simulink model "RealSimTemplate"  (R2019b)
settings: Solver=FixedStepAuto  StartTime=0.0  StopTime=200  FixedStep=0.001  RelTol=1e-3
settings Model: Creator=y0n  LastModifiedBy=y0n
settings DataIOCC: SaveOutput=off  SignalLogging=off  DSMLogging=off  SaveTime=off  ReturnWorkspaceOutputsName=VehicleOut
settings DebuggingCC: AlgebraicLoopMsg=none  UnderSpecifiedDimensionMsg=error
settings SFSimCC: CustomCodeUndefinedFunction=UseInterfaceOnly

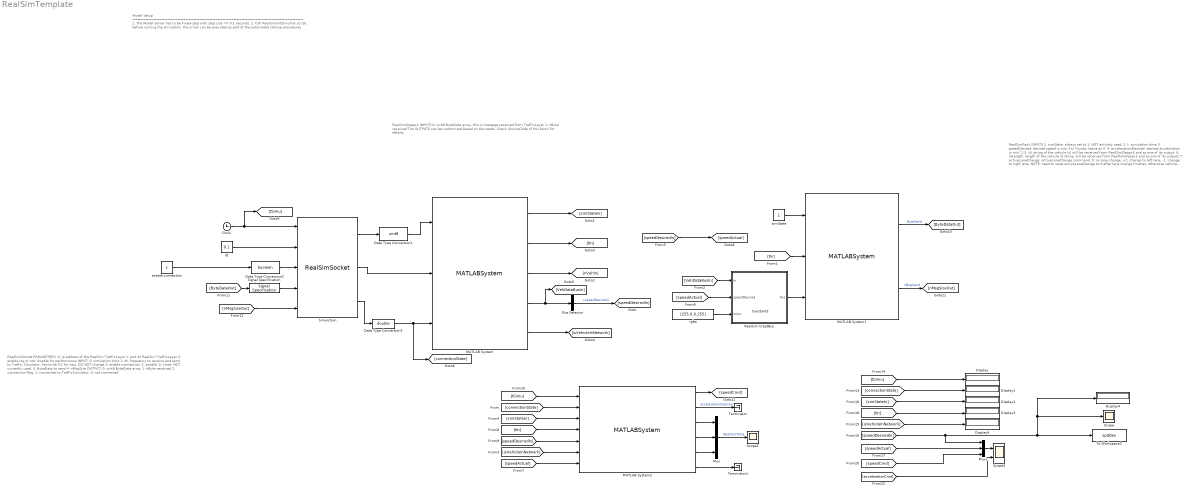
== system RealSimTemplate ==
  note: Model Setup
      | ================================================================
      | 1. The Model Solver has to be Fixed-step with step size <= 0.1 seconds.
      | 2. Call RealSimInitSimulink script before running the simulation. the script can be executed as part of the automated startup procedures.
  note: RealSimSocket
      | PARAMETERS:
      | 0: ip address of the RealSim TrafficLayer
      | 1: port to RealSim TrafficLayer
      | 2: enable log or not, disable for performance
      | INPUT:
      | 0: simulation time
      | 1: dt, frequency to receive and send to Traffic Simulator, has to be 0.1 for now, DO NOT change
      | 2: enable connection, 1: enable, 0: close. NOT currently used.
      | 3: ByteData to send
      | 4: nMsgSize
      |
      | OUTPUT:
      | 0: uint8 ByteData array
      | 1: nByte received
      | 2: connection flag, 1: connected to TrafficSimulator, 0: not connected
  note: RealSimPack
      | INPUTS
      | 1. simState: always set to 1. NOT actively used.
      | 2. t: simulation time
      | 3. speedDesired: desired speed in m/s, For Toyota, leave as 0.
      | 4. accelerationDesired: desired acceleration in m/s^2
      | 5. id: string of the vehicle id, will be received from RealSimDepack and as one of its output.
      | 6. idLength: length of the vehicle id string, will be received from RealSimDepack and as one of its outputs
      | 7: activeLaneChange: activeLaneChange command, 0: no lane change, +1: change to left lane, -1: change to right lane. NOTE: need to reset activeLaneChange to 0 after lane change finishes, otherwise vehicle will keep making lane change. Will receive 0 activeLaneChangeFdbk from RealSimDepack when lane change finishes.
      |
      | NOTE 1: Currently, only speedDesired and/or accelerationDesired can be sent to VISSIM/SUMO. The data format receive and send are the same so other mesage fields of the send data are irrelevant and can be set to empty or zero.
      |
      | NOTE 2: if select both speedDesired and accelerationDesired
      | in config.yaml, then only accelerationDesired will be used
      | to control vehicles in TrafficSimulator. if only one of
      | speedDesired and accelerationDesired selected in
      | config.yaml, then the one selected will be used for
      | control, the other input can be leave as 0.
      |
      | NOTE 3: for VISSIM, speedDesired or accelerationDesired will be the control command 0.2 seconds in the future.
      |
      | OUTPUTS
      | 1.ByteData: bytes vector that will be sent to TrafficSimualtor
      | 2.nMsgSize: size of bytes to be sent
  note: RealSimDepack
      | INPUTS
      | 0: uint8 ByteData array, this is message received from TrafficLayer
      | 1: nByte received
      |
      | The OUTPUTS can be customized based on the needs. Check SourceCode of this block for details.
  Bus Selector : BusSelector  OutputSignals=speedDesired
  Clock : Clock
  Constant3 : Constant  Value=0
  Data Type Conversion1 : DataTypeConversion  OutDataTypeStr=uint8
  Data Type Conversion2 : DataTypeConversion  OutDataTypeStr=boolean
  Data Type Conversion3 : DataTypeConversion  OutDataTypeStr=double
  Display{,1..4,6} (6 alike) : Display
  MATLAB System : MATLABSystem  System=RealSimDepack  OutputBusName=VehDataBus  VehicleMessageFieldDefInputVec=VehicleMessageFieldDefInputVec  SimulateUsing=Code generation
      mask Type: RealSimDepack
      mask Display:
      | disp('RealSimDepack');
      | port_label('input',1,'ByteData');
      | port_label('input',2,'nByte');
      | port_label('input',3,'connectionState');
      | port_label('output',1,'simState');
      | port_label('output',2,'t');
      | port_label('output',3,'nVeh');
      | port_label('output',4,'VehDataBus');
      | port_label('output',5,'isVehicleInNetwork');
  MATLAB System1 : MATLABSystem  System=RealSimPack  VehicleMessageFieldDefInputVec=VehicleMessageFieldDefInputVec  SimulateUsing=Code generation
      mask Type: RealSimPack
      mask Display:
      | disp('RealSimPack');
      | port_label('input',1,'simState');
      | port_label('input',2,'t');
      | port_label('input',3,'VehDataBus');
      | port_label('output',1,'ByteData');
      | port_label('output',2,'nMsgSize');
  MATLAB System2 : MATLABSystem  System=RealSimInterpSpeed  initialSpeed=RealSimPara.speedInit  speedLookAheadHorizon=RealSimPara.tLookahead  speedUpperBound=30  SimulateUsing=Code generation
      mask Type: RealSimInterpSpeed
      mask Display:
      | disp('RealSimInterpSpeed');
      | port_label('input',1,'simulationTime');
      | port_label('input',2,'connectionState');
      | port_label('input',3,'simState');
      | port_label('input',4,'timeReceive');
      | port_label('input',5,'speedReceive');
      | port_label('input',6,'isVehicleInNetwork');
      | port_label('input',7,'speedActual');
      | port_label('output',1,'speedLookAhead');
      | port_label('output',2,'accelerationDesired');
      | port_label('output',3,'timeSimulator');
      | port_label('output',4,'timeStepSimulator');
      | port_label('output',5,'timeStepTrigger');
      | port_label('output',6,'RealSimDelay');
  Mux : Mux  Inputs=3
  Mux1 : Mux  Inputs=3
  RealSim CreatBus : Subsystem
  S-Function : S-Function  FunctionName=RealSimSocket  Parameters=TrafficLayerIP, TrafficLayerPort, 0  SFunctionDeploymentMode=off  EnableBusSupport=off
  Scope : Scope
  Scope1 : Scope
  Scope3 : Scope  NumInputPorts=2
  Signal Specification : SignalSpecification  Dimensions=[200 1]
  Terminator : Terminator
  Terminator1 : Terminator
  To Workspace2 : ToWorkspace  VariableName=spdDes  SaveFormat=Structure With Time  SampleTime=-1
  dt : Constant  Value=0.1
  enable connection : Constant
  rgba : Constant  Value=[255,0,0,255]
  simState : Constant
  wires:
  dt/1 -> S-Function/2
  S-Function/1 -> Data Type Conversion1/1
  S-Function/2 -> MATLAB System/2
  Data Type Conversion1/1 -> MATLAB System/1
  enable connection/1 -> Data Type Conversion2/1
  Data Type Conversion2/1 -> S-Function/3
  S-Function/3 -> Data Type Conversion3/1
  MATLAB System/1 -> [simStateIn]
  Signal Specification/1 -> S-Function/4
  Bus Selector/1 -> [speedDesiredIn]  "<speedDesired>"
  MATLAB System/2 -> [tIn]
  MATLAB System/3 -> [nVehIn]
  MATLAB System/5 -> [isVehicleInNetwork]
  Data Type Conversion3/1 -> [connectionState], MATLAB System/3
  MATLAB System/4 -> [VehDataBusIn], Bus Selector/1
  [speedDesiredIn] -> MATLAB System2/5
  [tIn] -> MATLAB System2/4
  [connectionState] -> MATLAB System2/2
  [isVehicleInNetwork] -> MATLAB System2/6
  [simStateIn] -> MATLAB System2/3
  [tSimu] -> MATLAB System2/1
  [speedDesiredIn] -> [speedActual]
  [speedActual] -> MATLAB System2/7
  Clock/1 -> [tSimu], S-Function/1
  [ByteDataOut] -> Signal Specification/1
  [nMsgSizeOut] -> S-Function/5
  MATLAB System2/1 -> [speedCmd]
  MATLAB System2/2 -> Terminator/1  "accelerationDesired"
  MATLAB System2/3 -> Mux/1
  MATLAB System2/4 -> Mux/2
  MATLAB System2/5 -> Mux/3
  Mux/1 -> Scope1/1  "RealSimTime"
  MATLAB System2/6 -> Terminator1/1
  rgba/1 -> RealSim CreatBus/3(color)
  [tIn] -> MATLAB System1/2
  RealSim CreatBus/1(Out) -> MATLAB System1/3
  [speedActual] -> RealSim CreatBus/2(speedDesired)
  MATLAB System1/2 -> [nMsgSizeOut]  "nMsgSend"
  MATLAB System1/1 -> [ByteDataOut]  "ByteSend"
  simState/1 -> MATLAB System1/1
  [VehDataBusIn] -> RealSim CreatBus/1(In)
  [accelerationCmd] -> Scope3/2
  Mux1/1 -> Scope3/1
  [speedActual] -> Mux1/2
  [tSimu] -> Display/1
  [speedDesiredIn] -> Display4/1, Scope/1, To Workspace2/1, Mux1/1
  [speedCmd] -> Mux1/3
  [connectionState] -> Display1/1
  [tIn] -> Display3/1
  [simStateIn] -> Display2/1
  [isVehicleInNetwork] -> Display6/1

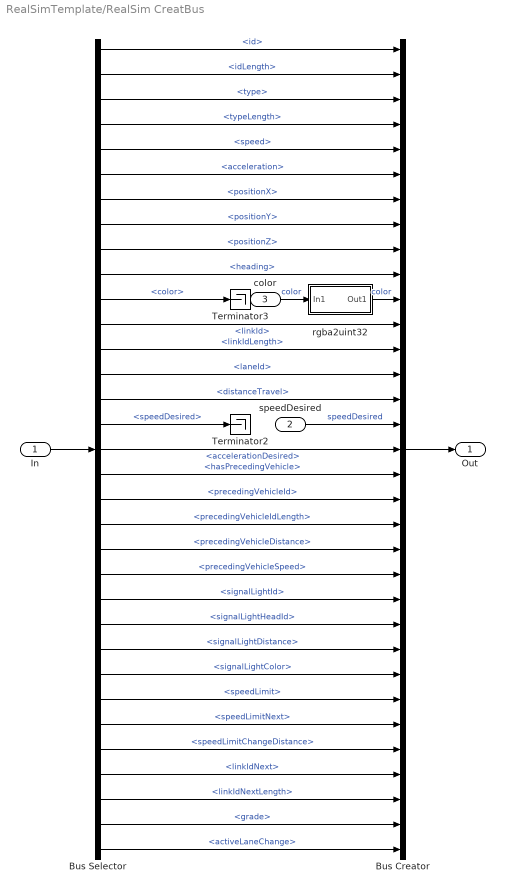
== system RealSimTemplate/RealSim CreatBus ==
  In : Inport
  speedDesired : Inport  Port=2
  color : Inport  Port=3
  Bus Creator : BusCreator  Inputs=33  OutDataTypeStr=Bus: VehDataBus
  Bus Selector : BusSelector  OutputSignals=id,idLength,type,typeLength,speed,acceleration,positionX,positionY,positionZ,heading,color,linkId,linkIdLength,laneId,distanceTravel,speedDesired,accelerationDesired,hasPrecedingVehicle,precedingVehicleId,precedingVehicleIdLength,precedingVehicleDistance,precedingVehicleSpeed,signalLightId,signalLightHeadId,signalLightDistance,signalLightColor,speedLimit,speedLimitNext,speedLimitChangeDistance,linkIdNext,linkIdNextLength,grade,activeLaneChange
  Terminator2 : Terminator
  Terminator3 : Terminator
  rgba2uint32 : Subsystem
  Out : Outport
  wires:
  In/1 -> Bus Selector/1
  Bus Creator/1 -> Out/1
  Bus Selector/1 -> Bus Creator/1  "<id>"
  Bus Selector/2 -> Bus Creator/2  "<idLength>"
  Bus Selector/3 -> Bus Creator/3  "<type>"
  Bus Selector/4 -> Bus Creator/4  "<typeLength>"
  Bus Selector/5 -> Bus Creator/5  "<speed>"
  Bus Selector/6 -> Bus Creator/6  "<acceleration>"
  Bus Selector/7 -> Bus Creator/7  "<positionX>"
  Bus Selector/8 -> Bus Creator/8  "<positionY>"
  Bus Selector/9 -> Bus Creator/9  "<positionZ>"
  Bus Selector/10 -> Bus Creator/10  "<heading>"
  Bus Selector/11 -> Terminator3/1  "<color>"
  Bus Selector/12 -> Bus Creator/12  "<linkId>"
  Bus Selector/13 -> Bus Creator/13  "<linkIdLength>"
  Bus Selector/14 -> Bus Creator/14  "<laneId>"
  Bus Selector/15 -> Bus Creator/15  "<distanceTravel>"
  Bus Selector/16 -> Terminator2/1  "<speedDesired>"
  Bus Selector/17 -> Bus Creator/17  "<accelerationDesired>"
  Bus Selector/18 -> Bus Creator/18  "<hasPrecedingVehicle>"
  Bus Selector/19 -> Bus Creator/19  "<precedingVehicleId>"
  Bus Selector/20 -> Bus Creator/20  "<precedingVehicleIdLength>"
  Bus Selector/21 -> Bus Creator/21  "<precedingVehicleDistance>"
  Bus Selector/22 -> Bus Creator/22  "<precedingVehicleSpeed>"
  Bus Selector/23 -> Bus Creator/23  "<signalLightId>"
  Bus Selector/24 -> Bus Creator/24  "<signalLightHeadId>"
  Bus Selector/25 -> Bus Creator/25  "<signalLightDistance>"
  Bus Selector/26 -> Bus Creator/26  "<signalLightColor>"
  Bus Selector/27 -> Bus Creator/27  "<speedLimit>"
  Bus Selector/28 -> Bus Creator/28  "<speedLimitNext>"
  Bus Selector/29 -> Bus Creator/29  "<speedLimitChangeDistance>"
  Bus Selector/30 -> Bus Creator/30  "<linkIdNext>"
  Bus Selector/31 -> Bus Creator/31  "<linkIdNextLength>"
  Bus Selector/32 -> Bus Creator/32  "<grade>"
  Bus Selector/33 -> Bus Creator/33  "<activeLaneChange>"
  speedDesired/1 -> Bus Creator/16  "speedDesired"
  color/1 -> rgba2uint32/1(In1)  "color"
  rgba2uint32/1(Out1) -> Bus Creator/11  "color"

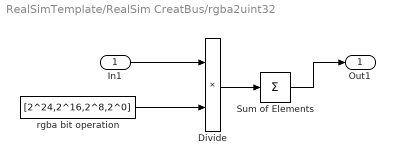
== system RealSimTemplate/RealSim CreatBus/rgba2uint32 ==
  In1 : Inport
  Divide : Product  Inputs=**
  Sum of Elements : Sum  Inputs=+
  rgba bit operation : Constant  Value=[2^24,2^16,2^8,2^0]
  Out1 : Outport
  wires:
  Divide/1 -> Sum of Elements/1
  In1/1 -> Divide/1
  rgba bit operation/1 -> Divide/2
  Sum of Elements/1 -> Out1/1
